simulink model "cannon3_group03"  (R2021a)
settings: Solver=VariableStepAuto  StartTime=0.0  StopTime=25  RelTol=1e-3
settings Model: Creator=zeoliam  LastModifiedBy=gasiewca

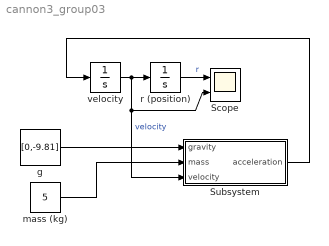
== system cannon3_group03 ==
  Scope : Scope  NumInputPorts=2
  Subsystem : Subsystem
  g : Constant  Value=[0,-9.81]
  mass (kg) : Constant  Value=5
  r (position) : Integrator  InitialCondition=[0 0]
  velocity : Integrator  InitialCondition=[100 100]
  wires:
  mass (kg)/1 -> Subsystem/2(mass)
  velocity/1 -> Subsystem/3(velocity), Scope/2, r (position)/1  "velocity"
  r (position)/1 -> Scope/1  "r"
  g/1 -> Subsystem/1(gravity)
  Subsystem/1(acceleration) -> velocity/1

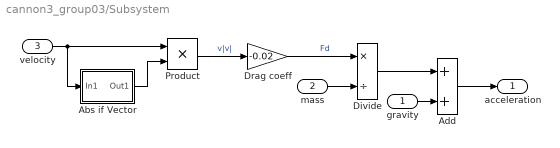
== system cannon3_group03/Subsystem ==
  gravity : Inport
  mass : Inport  Port=2
  velocity : Inport  Port=3
  Abs if Vector : Subsystem
  Add : Sum
  Divide : Product  Inputs=*/
  Drag coeff : Gain  Gain=-0.02
  Product : Product
  acceleration : Outport
  wires:
  velocity/1 -> Abs if Vector/1(In1), Product/1
  Product/1 -> Drag coeff/1  "v|v|"
  Drag coeff/1 -> Divide/1  "Fd"
  mass/1 -> Divide/2
  Divide/1 -> Add/1
  gravity/1 -> Add/2
  Add/1 -> acceleration/1
  Abs if Vector/1(Out1) -> Product/2

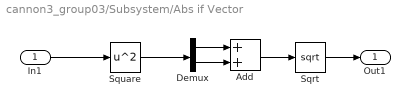
== system cannon3_group03/Subsystem/Abs if Vector ==
  In1 : Inport
  Add : Sum
  Demux : Demux  Outputs=2
  Sqrt : Sqrt  SaturateOnIntegerOverflow=on
  Square : Math  Operator=square  SaturateOnIntegerOverflow=on
  Out1 : Outport
  wires:
  In1/1 -> Square/1
  Square/1 -> Demux/1
  Demux/1 -> Add/1
  Demux/2 -> Add/2
  Add/1 -> Sqrt/1
  Sqrt/1 -> Out1/1
